simulink model "ORR_Part5"  (R2024b)
settings: Solver=VariableStepAuto  StartTime=0.0  StopTime=tspan  RelTol=1e-3
values from neighbouring files (symbols this model uses):
  E_b_ECI_0 = [phi_b_eci_0; theta_b_eci_0; psi_b_eci_0]    [Final_4.m]    (also in Part3_Disturbance.m = C2EulerAngles(C_b_ECI_0); Part_3_Disturbance_ORR.m = C2euler(C_b_eci_0); Part_5_ORR.m = C2euler(C_b_eci_0))
  J = n.sat.I    [Part5_TorqueFreeMotion_SS.m]    (also in Part_2_TorqueFreeMotion_Orr.m = [812.0396         0         0; Part_5_ORR.m = [d.Ixx, d.Ixy, d.Ixz;         d.Ixy, d.Iyy, d.Iyz;         d)
  Kd = J/ts    [Part5_TorqueFreeMotion_SS.m]    (also in Part_5_ORR.m = J*eye(3)*2*zeta*wn; SS_Part6Script.m = 2*zeta*wn*I_tot)
  Kp = zeros(3)    [Part5_TorqueFreeMotion_SS.m]    (also in Part_5_ORR.m = 2*J*eye(3)*wn^2; SS_Part6Script.m = 2*wn^2*I_tot)
  q_b_ECI_0 = q_b_ECI_0(:)    [Final_4.m]    (also in Part3_Disturbance.m = C2quat(C_b_ECI_0); Part_3_Disturbance_ORR.m = C2quat(C_b_eci_0); Part_5_ORR.m = C2quat(C_b_eci_0))
  q_c = [E_c; sqrt(1 - norm(E_c)^2)]    [Part_5_ORR.m]
  T_d = 0    [ORR_part4_script.m]    (also in Part5_TorqueFreeMotion_SS.m = [0; 0; 0]; Part_5_ORR.m = [0; 0; 0])
  w_b_ECI_0 = w_b_ECI_0(:)    [Final_3.m]    (also in Final_4.m = [0.001; -0.001; 0.002]; ORR_part4_script.m = [0.001; -0.001; 0.002]; Part3_Disturbance.m = [0.001; -0.001; 0.002]; Part_3_Disturbance_ORR.m = [0.001; -0.001; 0.002])
settings Model: Creator=haile  LastModifiedBy=haile

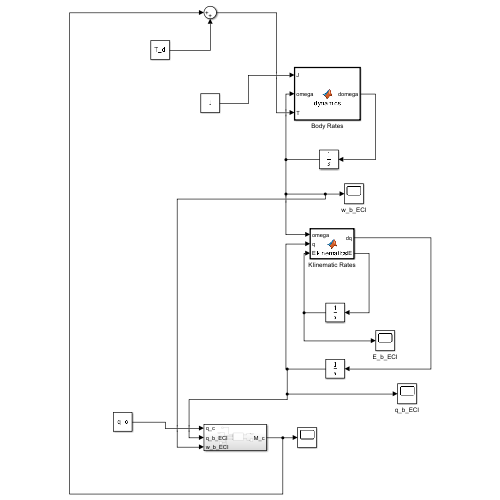
[thumbnail: Simulink's stored preview of the top-level diagram]
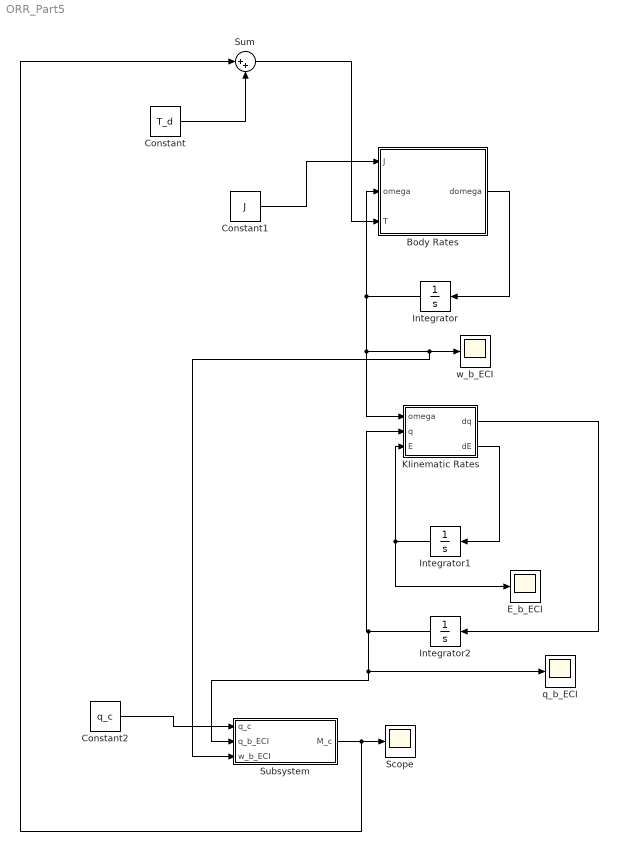
== system ORR_Part5 ==
  Body Rates : MATLAB Function  TreatAsAtomicUnit=on
  Constant : Constant  Value=T_d
  Constant1 : Constant  Value=J
  Constant2 : Constant  Value=q_c
  E_b_ECI : Scope
  Integrator : Integrator  InitialCondition=w_b_ECI_0
  Integrator1 : Integrator  InitialCondition=E_b_ECI_0
  Integrator2 : Integrator  InitialCondition=q_b_ECI_0
  KIinematic Rates : MATLAB Function  TreatAsAtomicUnit=on
  Scope : Scope
  Subsystem : Subsystem
  Sum : Sum  Inputs=|++
  q_b_ECI : Scope
  w_b_ECI : Scope
  wires:
  Constant/1 -> Sum/2
  Body Rates/1(domega) -> Integrator/1
  Integrator/1 -> Subsystem/3(w_b_ECI), w_b_ECI/1, KIinematic Rates/1(omega), Body Rates/2(omega)
  KIinematic Rates/2(dE) -> Integrator1/1
  Integrator1/1 -> E_b_ECI/1, KIinematic Rates/3(E)
  KIinematic Rates/1(dq) -> Integrator2/1
  Integrator2/1 -> Subsystem/2(q_b_ECI), q_b_ECI/1, KIinematic Rates/2(q)
  Constant2/1 -> Subsystem/1(q_c)
  Sum/1 -> Body Rates/3(T)
  Constant1/1 -> Body Rates/1(J)
  Subsystem/1(M_c) -> Sum/1, Scope/1

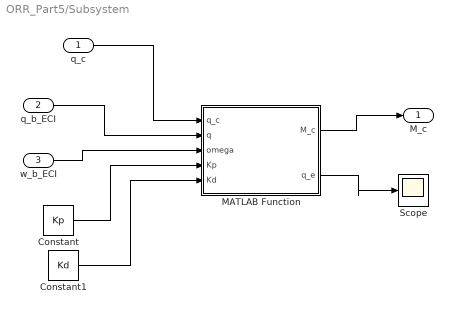
== system ORR_Part5/Subsystem ==
  q_c : Inport
  q_b_ECI : Inport  Port=2
  w_b_ECI : Inport  Port=3
  Constant : Constant  Value=Kp
  Constant1 : Constant  Value=Kd
  MATLAB Function : MATLAB Function  TreatAsAtomicUnit=on
  Scope : Scope
  M_c : Outport
  wires:
  q_c/1 -> MATLAB Function/1(q_c)
  q_b_ECI/1 -> MATLAB Function/2(q)
  w_b_ECI/1 -> MATLAB Function/3(omega)
  Constant/1 -> MATLAB Function/4(Kp)
  Constant1/1 -> MATLAB Function/5(Kd)
  MATLAB Function/1(M_c) -> M_c/1
  MATLAB Function/2(q_e) -> Scope/1

== matlab function ORR_Part5/KIinematic Rates ==
  data: omega input; dq output; q input; E input; dE output
function [dq, dE] = kinematics(omega, q, E)

    I = [1 0 0
        0 1 0
        0 0 1];

    omega = omega(:);
    E = E(:);
    q = q(:);
   
    theta_x = E(1);
    theta_y = E(2);
    %theta_z = e(3); not necessary in calculations

    epsilon = q(1:3);
    eta = q(4);

    C21 = [cos(theta_y) sin(theta_x) * sin(theta_y) cos(theta_x) * sin(theta_y)
      0 cos(theta_x) * cos(theta_y) -sin(theta_x) * cos(theta_y)
      0 sin(theta_x) cos(theta_x)];
    
    epsilon_dot = 0.5 * (eta * I * omega + cross(epsilon, omega));
    eta_dot = -0.5 * epsilon.' * omega;
    dq = [epsilon_dot; eta_dot];

    dE = (1 / cos(theta_y)) * C21 * omega;

end

== matlab function ORR_Part5/Body Rates ==
  data: domega output; J input; omega input; T input
function domega = dynamics(J, omega, T)

T = T(:);
omega = omega(:);

% step 1: use eulers equation to calculate angular velocity change
domega = inv(J) * (T - cross(omega, J*omega));


end

== matlab function ORR_Part5/Subsystem/MATLAB Function ==
  data: q_c input; M_c output size=[3 1]; q input; omega input; Kp input; Kd input; q_e output
function [M_c, q_e] = control_law(q_c, q, omega, Kp, Kd)
%#codegen

q_c = q_c(:);
q = q(:);
omega = omega(:);

q_e = quatMult(quatConjugate(q_c), q);
Mc = -Kp*q_e(1:3,1) - Kd*omega;



function quatconj = quatConjugate(q)

    quatconj = [-q(1:3);
        q(4)];

end

function w = quatMult(p, q)

    e_p = p(1:3);
    e_q = q(1:3);
    eta_p = p(4);
    eta_q = q(4);

    w = [eta_p*e_q + eta_q*e_p + vcross(e_p)*e_q;
        eta_p*eta_q - e_p'*e_q];
end

end
